simulink model "fff"  (R2017b)
settings: Solver=VariableStepAuto  StartTime=0.0  StopTime=10.0  RelTol=1e-3
settings Model: Creator=Salar  LastModifiedBy=Salar

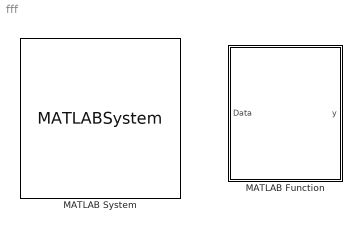
== system fff ==
  MATLAB Function : MATLAB Function  TreatAsAtomicUnit=on
  MATLAB System : MATLABSystem  System=HTFE  ChannelBandwidth=CBW20  SymbolTimingThreshold=1  OFDMSymbolOffset=.75  SimulateUsing=Code generation
      mask Type: HTFE
      mask Display:
      | disp('HTFE');
      | port_label('input',1,'x');
      | port_label('output',1,'validPacket');
      | port_label('output',2,'cfgNonHT');
      | port_label('output',3,'rxNonHTData');
      | port_label('output',4,'chanEst');
      | port_label('output',5,'noiseVarEst');
      | port_label('output',6,'data');
      | port_label('output',7,'cfo_est');
      | port_label('output',8,'channel_est');

== matlab function fff/MATLAB Function ==
  data: Data input; y output
function y = Channel_CFO_Estimation(Data)
        
    % Setup Front-End Packet Synchronizer
WLANFrontEnd = HTFE('ChannelBandwidth', 'CBW20');  




y = u;
